simulink model "LinearizedModel"  (R2023a)
settings: Solver=VariableStepAuto  StartTime=0.0  StopTime=0.1  RelTol=1e-3
InitFcn:
  | ROBLab2
undefined symbols (not defined in the file or in its folder): A, B, qdq_0
settings Model: Creator=dervint  LastModifiedBy=dervint

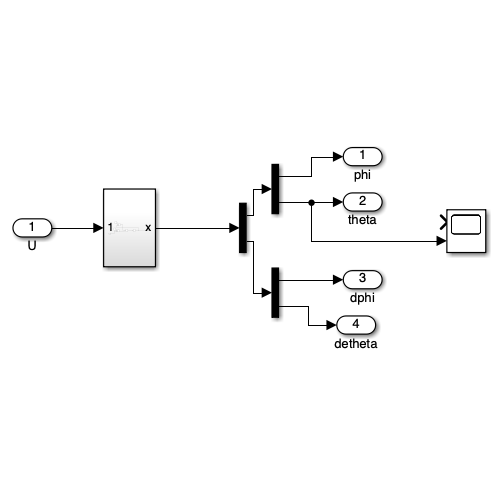
[thumbnail: Simulink's stored preview of the top-level diagram]
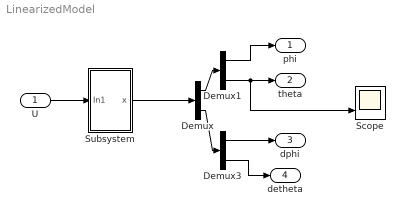
== system LinearizedModel ==
  U : Inport
  Demux : Demux  Outputs=2
  Demux1 : Demux  Outputs=2
  Demux3 : Demux  Outputs=2
  Scope : Scope  NumInputPorts=2
  Subsystem : Subsystem
  phi : Outport
  theta : Outport  Port=2
  dphi : Outport  Port=3
  detheta : Outport  Port=4
  wires:
  Demux/1 -> Demux1/1
  Demux/2 -> Demux3/1
  Demux1/2 -> Scope/2, theta/1
  Demux1/1 -> phi/1
  Demux3/1 -> dphi/1
  Demux3/2 -> detheta/1
  U/1 -> Subsystem/1(In1)
  Subsystem/1(x) -> Demux/1

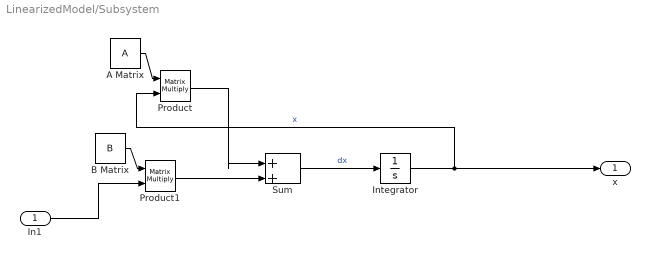
== system LinearizedModel/Subsystem ==
  In1 : Inport
  A Matrix : Constant  Value=A  VectorParams1D=off
  B Matrix : Constant  Value=B  VectorParams1D=off
  Integrator : Integrator  InitialCondition=qdq_0
  Product : Product  Inputs=**  Multiplication=Matrix(*)
  Product1 : Product  Inputs=**  Multiplication=Matrix(*)
  Sum : Sum  Inputs=|++
  x : Outport
  wires:
  Product/1 -> Sum/1
  Integrator/1 -> x/1, Product/2  "x"
  A Matrix/1 -> Product/1
  B Matrix/1 -> Product1/1
  Sum/1 -> Integrator/1  "dx"
  In1/1 -> Product1/2
  Product1/1 -> Sum/2
